simulink model "FooBlink"  (R2021a)
settings: Solver=FixedStepAuto  StartTime=0.0  StopTime=inf  RelTol=1e-6  EnableMultiTasking=on
InitFcn:
  | l = 0;
libraries: arduinolib x3, arduinosensorlib x1, simulink x1
settings Model: SILPILModeSetting=veronly  ExtModeTrigDuration=2  Creator=angelo  LastModifiedBy=angelo
settings OptimizationCC: EnhancedBackFolding=on  PassReuseOutputArgsAs=Individual arguments  ZeroExternalMemoryAtStartup=off  ZeroInternalMemoryAtStartup=off  MaxStackSize=64  OptimizeBlockOrder=speed  DifferentSizesBufferReuse=on  OptimizationCustomize=off  EfficientTunableParamExpr=on
settings DebuggingCC: ParameterTunabilityLossMsg=error
settings HardwareCC: ProdBitPerInt=16  ProdBitPerPointer=16  ProdBitPerSizeT=16  ProdBitPerPtrDiffT=16  ProdLargestAtomicFloat=None  ProdWordSize=8  ProdHWDeviceType=Atmel->AVR
settings SFSimCC: MATLABDynamicMemAlloc=off
settings RTWCC: SystemTargetFile=ert.tlc  HardwareBoard=Arduino Mega 2560  TemplateMakefile=ert_default_tmf  Toolchain=Arduino AVR  BuildConfiguration=Faster Runs
settings CodeAppCC: ForceParamTrailComments=on  IgnoreCustomStorageClasses=off  OperatorAnnotations=on  SimulinkDataObjDesc=on  SFDataObjDesc=on  InsertBlockDesc=on
settings ERTTargetCC: SupportContinuousTime=on  SupportVariableSizeSignals=on  ExtModeStaticAllocSize=2048

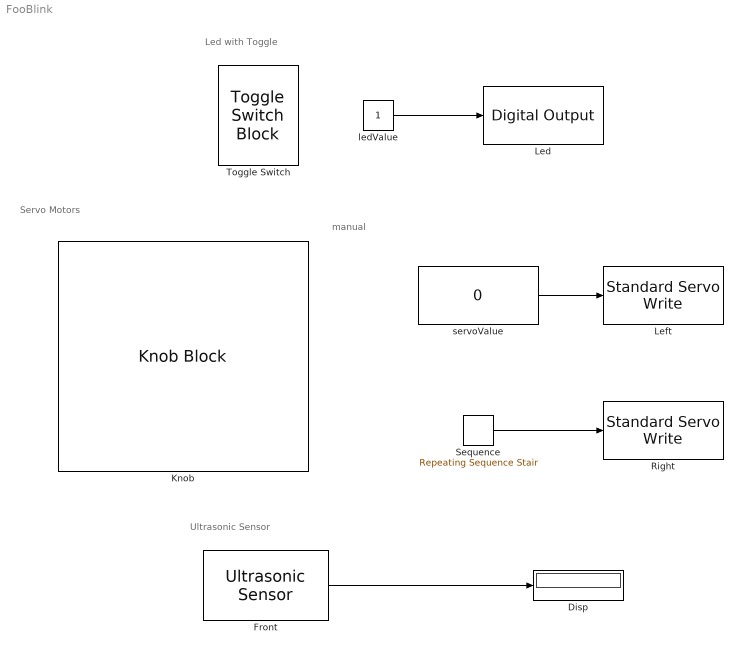
== system FooBlink ==
  note: manual
  note: Led with Toggle
  note: Ultrasonic Sensor
  note: Servo Motors
  Disp : Display
  Front : arduinosensorlib/Ultrasonic Sensor  NumSignalPins=2  TrigPin=3  EchoPin=4  SignalPin=3  SampleTime_=0.1  blockPlatform=ARDUINO
      settings: SourceProductBaseCode=ARDUINO
  Knob : KnobBlock  ScaleMax=180
  Led : arduinolib/Digital Output  pinNumber=7  Direction=output  blockPlatform=arduino
  Left : arduinolib/Standard Servo Write  pinNumber=9  ServoIndex=0  blockPlatform=ARDUINO
  Right : arduinolib/Standard Servo Write  pinNumber=2  ServoIndex=1  blockPlatform=ARDUINO
  Sequence : simulink/Sources/Repeating Sequence Stair  OutValues=[0 45 90 180 90 45 0]  tsamp=1  OutMin=[]  OutMax=[]  OutDataTypeStr=double  OutputDataTypeScalingMode=double  OutDataType=fixdt(0,8)  ConRadixGroup=Best Precision: Vector-wise  OutScaling=2^-12
  Toggle Switch : ToggleSwitchBlock
      settings: Values={{'Off', 'On'}, [0 1]}
  ledValue : Constant
  servoValue : Constant  Value=0
  wires:
  ledValue/1 -> Led/1
  Front/1 -> Disp/1
  servoValue/1 -> Left/1
  Sequence/1 -> Right/1
